simulink model "sim_all_2019b"  (R2019b)
settings: Solver=VariableStepAuto  StartTime=0.0  StopTime=2000  RelTol=1e-3
undefined symbols (not defined in the file or in its folder): a1, a2, alpha1, alpha2, cornerA, cornerB, cornerC, cornerD, ctrl_clockwise, ctrl_int_bound_or, ctrl_int_bound_pos, ctrl_k_or, ctrl_k_pos, ctrl_Ki_vel, ctrl_Kp_v_pos, ctrl_Kp_vel, ctrl_TAM, ctrl_Ts, ctrl_va_uncontrolled, ctrl_vel_uncontrolled, D, dead_zone_limit, depth, DiscIntNeverNeededParam, distanceFromWall, initInspectedSide, initPoint, mod_A, mod_Cd_F, mod_Cd_M, mod_eta_init, mod_g, mod_h0, mod_Ixx, mod_Iyy, mod_Izz, mod_Kp_dot, mod_lat0, mod_lon0, mod_m, mod_Mq_dot, mod_ni_init, mod_Nr_dot, mod_p1, mod_p2, mod_p3, mod_p4, mod_p5, mod_p6, mod_R, mod_Rm, mod_t1, mod_t2, mod_t3, mod_t4, mod_t5, mod_t6, mod_W, mod_Xu_dot, mod_Yv_dot ... (+53)
libraries: simulink x8, cstblocks x6, simulink_extras x1
(part 5 of 6)

== matlab function sim_all_2019b/Model/Vehicle Model/P3/Propeller3 ==
  data: n3 input; T3 output; V3 input; D parameter; omega parameter; a1 parameter; a2 parameter; alpha1 parameter; alpha2 parameter
function T3 = thrusterModel(n3, V3, D, omega, a1, a2, alpha1, alpha2)

Va3 = (1-omega) * V3;     % Advancement velocity at the propeller
J0 = Va3/(n3*D);          % Advancement Coefficient

if J0 > -alpha1/alpha2  % Out of linearity domain (right side)
    T3 = 0;              % A null generated thrust is assumed
    
elseif J0 < 0           % Out of linearity domain (left side)
    T3 = a1*abs(n3)*n3;    % Bollard thrust is assumed

else                    % Within the linearity domain
    T3 = a1*abs(n3)*n3 - a2*abs(n3)*V3;
end

== matlab function sim_all_2019b/Model/Vehicle Model/P4/Propeller4 ==
  data: n4 input; T4 output; V4 input; D parameter; omega parameter; a1 parameter; a2 parameter; alpha1 parameter; alpha2 parameter
function T4 = thrusterModel(n4, V4, D, omega, a1, a2, alpha1, alpha2)

Va4 = (1-omega) * V4;     % Advancement velocity at the propeller
J0 = Va4/(n4*D);          % Advancement Coefficient

if J0 > -alpha1/alpha2  % Out of linearity domain (right side)
    T4 = 0;              % A null generated thrust is assumed
    
elseif J0 < 0           % Out of linearity domain (left side)
    T4 = a1*abs(n4)*n4;    % Bollard thrust is assumed

else                    % Within the linearity domain
    T4 = a1*abs(n4)*n4 - a2*abs(n4)*V4;
end

== matlab function sim_all_2019b/Model/Vehicle Model/P5/Propeller5 ==
  data: n5 input; T5 output; V5 input; D parameter; omega parameter; a1 parameter; a2 parameter; alpha1 parameter; alpha2 parameter
function T5 = thrusterModel(n5, V5, D, omega, a1, a2, alpha1, alpha2)

Va5 = (1-omega) * V5;     % Advancement velocity at the propeller
J0 = Va5/(n5*D);          % Advancement Coefficient

if J0 > -alpha1/alpha2  % Out of linearity domain (right side)
    T5 = 0;              % A null generated thrust is assumed
    
elseif J0 < 0           % Out of linearity domain (left side)
    T5 = a1*abs(n5)*n5;    % Bollard thrust is assumed

else                    % Within the linearity domain
    T5 = a1*abs(n5)*n5 - a2*abs(n5)*V5;
end

== matlab function sim_all_2019b/Model/Vehicle Model/P6/Propeller6 ==
  data: n6 input; T6 output; V6 input; D parameter; omega parameter; a1 parameter; a2 parameter; alpha1 parameter; alpha2 parameter
function T6 = thrusterModel(n6, V6, D, omega, a1, a2, alpha1, alpha2)

Va6 = (1-omega) * V6;     % Advancement velocity at the propeller
J0 = Va6/(n6*D);          % Advancement Coefficient

if J0 > -alpha1/alpha2  % Out of linearity domain (right side)
    T6 = 0;              % A null generated thrust is assumed
    
elseif J0 < 0           % Out of linearity domain (left side)
    T6 = a1*abs(n6)*n6;    % Bollard thrust is assumed

else                    % Within the linearity domain
    T6 = a1*abs(n6)*n6 - a2*abs(n6)*V6;
end

== matlab function sim_all_2019b/Model/Vehicle Model/TAM ==
  data: T1 input; tau output; T2 input; T3 input; T4 input; T5 input; T6 input; eta input; mod_R parameter; mod_z_cm parameter
function tau = fcn (T1, T2, T3, T4, T5, T6, eta, mod_R, mod_z_cm)

% Si definisce il vettore delle forze e dei momenti applicati al veicolo al 
% variare dei propulsori immersi o emersi, si assume che i propulsori non 
% funzionino se utilizzati fuori dall'acqua. Si assume inoltre che il
% veicolo esca fuori dall'acqua orizzontalmente (con angoli di pitch e roll
% nulli).

z = eta(3);

% Veicolo completamente immerso, tutti i propulsori funzionano.
if (z >= (mod_R+mod_z_cm)) 
    tau1 = T1 + T2;
    tau2 = T3 + T4;
    tau3 = T5 + T6;
    tau4 = ((-(mod_R+mod_z_cm))*T3) + ((mod_R+mod_z_cm)*T4);
    tau5 = (-mod_R*T5) + (mod_R*T6);
    tau6 = (-mod_R*T1) + (mod_R*T2);
    
% Veicolo emerso in un range che va al dall'estremo superiore fino al 
% centro di massa (il centro di massa è ancora immerso), funzionano tutti i 
% propulsori tranne P4.
elseif (z >= 0 && z < (mod_R+mod_z_cm)) 
    tau1 = T1 + T2;
    tau2 = T3;
    tau3 = T5 + T6;
    tau4 = ((-(mod_R+mod_z_cm))*T3);
    tau5 = (-mod_R*T5) + (mod_R*T6);
    tau6 = (-mod_R*T1) + (mod_R*T2);

% Veicolo immerso in un range che va dall'estremo inferiore fino al centro 
% di massa (il centro di massa è emerso), funziona solo il propulsore P3.
elseif (z >= -(mod_R+mod_z_cm) && z < 0)
    tau1 = 0;
    tau2 = T3;
    tau3 = 0;
    tau4 = ((-(mod_R+mod_z_cm))*T3);
    tau5 = 0;
    tau6 = 0;

% Veicolo completamente emerso, nessun propulsore funziona.
else
    tau1 = 0;
    tau2 = 0;
    tau3 = 0;
    tau4 = 0;
    tau5 = 0;
    tau6 = 0;
end

tau = [tau1; tau2; tau3; tau4; tau5; tau6];

== matlab function sim_all_2019b/Model/Vehicle Model/Thruster Velocity Computation ==
  data: V1 output; V2 output; V3 output; V4 output; V5 output; V6 output; ni_rel input; mod_p1 parameter; mod_p2 parameter; mod_p3 parameter; mod_p4 parameter; mod_p5 parameter; mod_p6 parameter; mod_t1 parameter; mod_t2 parameter; mod_t3 parameter; mod_t4 parameter; mod_t5 parameter; mod_t6 parameter
function [V1, V2, V3, V4, V5, V6] = fcn(ni_rel, mod_p1, mod_p2, mod_p3, mod_p4, mod_p5, mod_p6, mod_t1, mod_t2, mod_t3, mod_t4, mod_t5, mod_t6)

% Si spezza il vettore velocità relativa nella componente lineare e angolare:
ni1_rel = [ni_rel(1); ni_rel(2); ni_rel(3)];
ni2_rel = [ni_rel(4); ni_rel(5); ni_rel(6)];

% Si definiscono i vettori velocità dei propulsori: 
Vp1 = ni1_rel + cross(ni2_rel, mod_p1);
Vp2 = ni1_rel + cross(ni2_rel, mod_p2);
Vp3 = ni1_rel + cross(ni2_rel, mod_p3);
Vp4 = ni1_rel + cross(ni2_rel, mod_p4);
Vp5 = ni1_rel + cross(ni2_rel, mod_p5);
Vp6 = ni1_rel + cross(ni2_rel, mod_p6);

% Si proiettano tali velocità lungo le direzioni date dai versori:
V1 = dot(Vp1, mod_t1); 
V2 = dot(Vp2, mod_t2);
V3 = dot(Vp3, mod_t3);
V4 = dot(Vp4, mod_t4);
V5 = dot(Vp5, mod_t5);
V6 = dot(Vp6, mod_t6);

== matlab function sim_all_2019b/Model/Vehicle Model/seaCurrent from NED to body ==
  data: seaCurrent_Velocity output; eta input; seaCurrent parameter
function seaCurrent_Velocity = fcn(eta, seaCurrent)

phi = eta(4);
theta = eta(5); 
psi = eta(6);

% Si definisce la matrice di rotazione J1 che mappa la velocità lineare 
% della corrente in terna body nella velocità lineare della corrente in 
% terna NED: 
J1 = [ cos(psi)*cos(theta)   -sin(psi)*cos(phi) + (cos(psi)*sin(theta)*sin(phi))   (sin(psi)*sin(phi)) + (cos(psi)*cos(phi)*sin(theta));
       sin(psi)*cos(theta)   (cos(psi)*cos(phi)) + (sin(psi)*sin(theta)*sin(phi))  (-cos(psi)*sin(phi)) + (sin(psi)*sin(theta)*cos(phi));
      -sin(theta)             cos(theta)*sin(phi)                                   cos(theta)*cos(phi)                                  ];

% Si definisce la matrice J1 inversa in maniera tale da mappare la velocità
% della corrente in terna NED nella velocità lineare della corrente in
% terna body (essendo J1 una matrice di rotazione l'inversa coincide con la
% trasposta):
J1_inv = J1';

%si definisce la velocità della corrente espressa in terna Body
seaCurrent_body = J1_inv*seaCurrent;
seaCurrent_Velocity = [seaCurrent_body; 0; 0; 0];

== matlab function sim_all_2019b/Model/from NED to ECEF ==
  data: eta1 input; eta1_ECEF output; mod_lat0 parameter; mod_lon0 parameter; mod_h0 parameter
function eta1_ECEF = fcn(eta1, mod_lat0, mod_lon0, mod_h0)

eta1_ECEF = [0; 0; 0];

eta1_North = eta1(1);
eta1_East = eta1(2);
eta1_Down = eta1(3);

coder.extrinsic('evalin','wgs84Ellipsoid','ned2geodetic')

[lat_ECEF, lon_ECEF, h_ECEF] = ned2geodetic(eta1_North, eta1_East, eta1_Down, mod_lat0, mod_lon0, mod_h0, wgs84Ellipsoid);

eta1_ECEF = [lat_ECEF; lon_ECEF; h_ECEF];

== matlab function sim_all_2019b/Sensors/BLOCCO GYRO1/Subsystem/GEOD to NED ==
  data: Bias_G output; t input
function Bias_G  = fcn(t)
ramp=t*(3.8785e-05);
Bias_G=ramp;

== matlab function sim_all_2019b/Controller_mk4_v3/C_pos/abs_integrator2/Body2Ned ==
  data: x_b input size=[3 1]; x_n output size=[3 1]; or input
%% Da BODY a NED per integrazione assoluta
function x_n = body2ned(x_b,or)
C=zeros(3,3);
C=Cx(or(1))'*Cy(or(2))'*Cz(or(3))';
x_n = C*x_b;
end

== matlab function sim_all_2019b/Controller_mk4_v3/C_pos/abs_integrator2/Ned2Body1 ==
  data: x_n input size=[3 1]; x_b output size=[3 1]; or input
%% Da NED a BODY
function x_b = ned2body(x_n,or)
C=zeros(3,3);
C=Cx(or(1))'*Cy(or(2))'*Cz(or(3))';
x_b = C'*x_n;
end

== matlab function sim_all_2019b/Controller_mk4_v3/C_pos/abs_integrator1/Body2Ned ==
  data: x_b input size=[3 1]; x_n output size=[3 1]; or input
%% Da BODY a NED
function x_n = body2ned(x_b,or)
C=zeros(3,3);
C=Cx(or(1))'*Cy(or(2))'*Cz(or(3))';
x_n = C*x_b;
end

== matlab function sim_all_2019b/Controller_mk4_v3/C_pos/abs_integrator1/Ned2Body1 ==
  data: x_n input size=[3 1]; x_b output size=[3 1]; or input
%% Da NED a BODY
function x_b = ned2body(x_n,or)
C=zeros(3,3);
C=Cx(or(1))'*Cy(or(2))'*Cz(or(3))';
x_b = C'*x_n;
end

== matlab function sim_all_2019b/Controller_mk4_v3/C_vel/abs_integrator/Body2Ned ==
  data: x_b input size=[3 1]; x_n output size=[3 1]; or input
%% Da BODY a NED
function x_n = body2ned(x_b,or)
C=zeros(3,3);
C=Cx(or(1))'*Cy(or(2))'*Cz(or(3))';
x_n = C*x_b;
end

== matlab function sim_all_2019b/Controller_mk4_v3/C_vel/abs_integrator/Ned2Body1 ==
  data: x_n input size=[3 1]; x_b output size=[3 1]; or input
%% Da NED a BODY
function x_b = ned2body(x_n,or)
C=zeros(3,3);
C=Cx(or(1))'*Cy(or(2))'*Cz(or(3))';
x_b = C'*x_n;
end

== matlab function sim_all_2019b/Mission_supervisor_v3/Mission_Supervisor/Risalita/MATLAB Function ==
  data: delta_SOS input; delta_current_ris output; delta_stato_ris output; Pos_d output size=3; Dpp_d output; Dps_d output; Pos_s input; Dpp_s input; Orp_s input; Dps_s input; distanceFromWall parameter; Orp_d output; relativeDirection parameter; soglia_pos parameter; SOS parameter; Dps_fin input; soglia_SOS_pos_ris parameter; soglia_SOS_orp parameter; error_flag input; SOS_205 input; initPoint parameter; soglia_SOS_collisione parameter
function [delta_current_ris, delta_stato_ris, Pos_d, Dpp_d, Dps_d, Orp_d ] = Risalita(delta_SOS, Pos_s, Dpp_s, Orp_s, Dps_s, distanceFromWall, relativeDirection, soglia_pos, SOS, Dps_fin, soglia_SOS_pos_ris, soglia_SOS_orp, error_flag, SOS_205, initPoint, soglia_SOS_collisione)

    disp("Risalita");
    
    %% Unità di misura 
    
    % Pos_d, Pos_s, soglia_pos, initPoint                                                                      [deg,deg,m]
    % Orp_d, Orp_s, soglia_SOS_orp                                                                             [rad]
    % relativeDirection                                                                                        [deg]
    % Dpp_d, Dps_d, Dpp_s, Dps_s, Dps_fin, distanceFromWall, soglia_SOS_collisione_s, soglia_SOS_collisione    [m]

    %% Inizializzazione variabili
    
    delta_stato_ris = 0;
    
    pronti = false; 
    
    %% Preparazione dei riferimenti da fornire ai blocchi successivi
    
    % Posizione da raggiungere
    Pos_d = [nan; nan; initPoint(3)];
    
    % Distanza da mantenere
    Dpp_d = distanceFromWall;
    Dps_d = Dps_fin;
    
    % Orientazione da mantenere
    Orp_d = deg2rad(relativeDirection);
    
    % Transizione di stato effettiva
    delta_current_ris = 301 - delta_SOS;  
    
    
    %% Verifica
    
    % Verifica sull'orientazione rispetto alla parete
    if (abs(Orp_s - Orp_d) > soglia_SOS_orp)
        
        SOS = 1;
        disp("EMERGENZA: Rilevato errore nell'orientazione relativa da parete");
        
    end
                                                                            %******TEST******
                                                                            %test = 30;
    % In base al meccanismo del "gestore dell'emergenza" si distinguono due casi: 
    % uno in cui lo stato di Risalita viene attivato al termine di un 
    % pattugliamento corretto (la codifica dello stato precedente è pari a 205) 
    % ed uno se la transizione in questo stato è dovuta all'aver
    % intrapreso una manovra di emergenza (lo stato precedente è
    % inferiore a 205).
    
    % Si proviene da un pattugliamento senza emergenza e si verifica di 
    % effettuare la risalita nella posizione giusta
    if (delta_SOS == 205 && SOS_205 == 0)
        if (abs(Dpp_s - Dpp_d) > soglia_SOS_pos_ris || ...                                          
            abs(Dps_s - Dps_fin) > soglia_SOS_pos_ris)
             
            SOS = 1;
            disp("EMERGENZA: Avvicinamento eccessivo alla parete");
            
        end
    
    % Si proviene da una situazione di emergenza oppure l'emergenza avviene in
    % "risalita". Verifica di effettuare la risalita senza collisione
    % con le pareti
    elseif (delta_SOS < 205 || SOS_205 == 1)
        
        if (abs(Dpp_s - Dpp_d) > soglia_SOS_collisione || ...
            abs(Dps_s) < soglia_SOS_collisione)
       
            SOS = 1;
            disp("EMERGENZA: Avvicinamento eccessivo alla parete");
            
        end
        
    end
    
    if error_flag == 1
        disp("EMERGENZA: Errore segnalato dagli altri sottosistemi");
        SOS = 1;
    end
    
                                                                            %*****TEST******% 
                                                                            %Dps_fin = 8;

    % Si verifica di aver raggiunto la superficie
    if (SOS == 0 && ... 
        abs(Pos_s(3) - Pos_d(3)) < soglia_pos(3)) 
    
          pronti = true;
        
    end
    
    
    %% Decisione dello stato successivo
    
    if ((pronti == true && (delta_SOS < 205 || SOS_205 == 1) || ...
        (SOS == 1)))
           
           delta_stato_ris = 304 - 301; % Transizione nello stato finale a causa di emergenza
    else
        if pronti == true
            
            delta_stato_ris = 302 - 301; % Transizione eseguita correttamente
        end
    end
    % Si rimane nello stato corrente
     
end

== matlab function sim_all_2019b/Controller_mk4_v3/lld2Ned1 ==
  data: x_ecef input size=[3 1]; x_n output; cornerC parameter
%% Da LLD (stima posizione assoluta) a NED
function x_n = ToNed_Pos(x_ecef,cornerC)
x_n=zeros(3,1);
coder.extrinsic('evalin', 'wgs84Ellipsoid', 'geodetic2ned');
[pNorth,pEast,pDown] = geodetic2ned(x_ecef(1),x_ecef(2),x_ecef(3),cornerC(1),cornerC(2),0,wgs84Ellipsoid);
x_n=[pNorth;pEast;x_ecef(3)];

end

== matlab function sim_all_2019b/Sensors/Environment and Sensors Model3/MATLAB Function1 ==
  data: pos input; plane_AB input; plane_BC input; plane_CD input; plane_DA input; plane_W input; dist output; Roll input; Pitch input; Yaw input
function dist = inter(pos,plane_AB,plane_BC,plane_CD,plane_DA,plane_W,Roll,Pitch, Yaw)
Nc=3; %numero di campioni per 'croce' di raggio del cono
WBr=deg2rad(5); % ampiezza semifascio del sonar (fascio considerato di 10°)
dist2=zeros(3,3);
R=linspace(Roll-WBr,Roll+WBr,Nc);
P=Pitch;
Y=linspace(Yaw-WBr, Yaw+WBr,Nc);
for j=1:Nc  %costruisco la croce (doppia)
for i=1:Nc
    
R_x = [1        0              0; %roll
      0 cos(R(i))  sin(R(i));
      0 -sin(R(i)) cos(R(i))];
  
R_y = [cos(P) 0 -sin(P); %pitch
          0           1         0;
       sin(P) 0 cos(P)];
   
R_z = [cos(Y(j)) sin(Y(j)) 0; %yaw
      -sin(Y(j)) cos(Y(j)) 0;
          0                 0        1];
      
jaco = (R_z'*R_y');
jacob = jaco*R_x';

    versore_son_body = [0 1 0]';
    versore_son_NED = jacob*versore_son_body;         %versore terna NED sonar prua

    %imposto il sistema per trovare l'intersezione tra la retta con direzione
    %nota e uno dei piani delle pareti del bacino

    t_AB = -(pos(1)+plane_AB(2)*pos(2)+plane_AB(4))/(plane_AB(2)*versore_son_NED(2)+versore_son_NED(1));
    t_BC = -(pos(1)+plane_BC(2)*pos(2)+plane_BC(4))/(plane_BC(2)*versore_son_NED(2)+versore_son_NED(1));
    t_CD = -(pos(1)+plane_CD(2)*pos(2)+plane_CD(4))/(plane_CD(2)*versore_son_NED(2)+versore_son_NED(1));
    t_DA = -(pos(1)+plane_DA(2)*pos(2)+plane_DA(4))/(plane_DA(2)*versore_son_NED(2)+versore_son_NED(1));
    t_W = -(plane_W(3)*pos(3)/(plane_W(3)*versore_son_NED(3)+versore_son_NED(3)));
    
    
    if t_AB < 0
        t_AB = inf;
    end
    if t_BC < 0
        t_BC = inf;
    end
    if t_CD < 0
        t_CD = inf;
    end
    if t_DA < 0
        t_DA = inf;
    end
    if t_W < 0
        t_W = inf;
    end
           dist1 = min([t_AB t_BC t_CD t_DA t_W]);
           
           if dist1==t_W %se incontro l'acqua metto NaN nella misura delle distanze
               dist2(i,j)=NaN;
           else
               dist2(i,j)=dist1;
           end
           
end
end
    contr=isnan(dist2); %controlla la presenza di NaN nel vettore di misure
    sum1=sum(sum(contr)); % conta il numero di NaN presenti
    
    if sum1>4 %incontro un numero di Nan superiore a 4
        dist=NaN;
    else
        dist=mean(nanmean(dist2));
    end
end

== matlab function sim_all_2019b/Sensors/Environment and Sensors Model4/MATLAB Function1 ==
  data: pos input size=[3]; plane_AB input; plane_BC input; plane_CD input; plane_DA input; plane_W input; dist output; Roll input; Pitch input; Yaw input
function dist = inter(pos,plane_AB,plane_BC,plane_CD,plane_DA,plane_W,Roll,Pitch, Yaw)
Nc=3; %numero di campioni per 'croce' di raggio del cono=1
WBr=deg2rad(5); % ampiezza semifascio del sonar (fascio considerato di 10°)
dist2=zeros(3,3);
R=linspace(Roll-WBr,Roll+WBr,Nc);
P=Pitch;
Y=linspace(Yaw-WBr, Yaw+WBr,Nc);
for j=1:Nc  %costruisco la croce (doppia)
for i=1:Nc
    
R_x = [1        0              0; %roll
      0 cos(R(i))  sin(R(i));
      0 -sin(R(i)) cos(R(i))];
  
R_y = [cos(P) 0 -sin(P); %pitch
          0           1         0;
       sin(P) 0 cos(P)];
   
R_z = [cos(Y(j)) sin(Y(j)) 0; %yaw
      -sin(Y(j)) cos(Y(j)) 0;
          0                 0        1];
      
jaco = (R_z'*R_y');
jacob = jaco*R_x';

    versore_son_body = [0 -1 0]';
    versore_son_NED = jacob*versore_son_body;         %versore terna NED sonar prua

    %imposto il sistema per trovare l'intersezione tra la retta con direzione
    %nota e uno dei piani delle pareti del bacino

    t_AB = -(pos(1)+plane_AB(2)*pos(2)+plane_AB(4))/(plane_AB(2)*versore_son_NED(2)+versore_son_NED(1));
    t_BC = -(pos(1)+plane_BC(2)*pos(2)+plane_BC(4))/(plane_BC(2)*versore_son_NED(2)+versore_son_NED(1));
    t_CD = -(pos(1)+plane_CD(2)*pos(2)+plane_CD(4))/(plane_CD(2)*versore_son_NED(2)+versore_son_NED(1));
    t_DA = -(pos(1)+plane_DA(2)*pos(2)+plane_DA(4))/(plane_DA(2)*versore_son_NED(2)+versore_son_NED(1));
    t_W = -(plane_W(3)*pos(3)/(plane_W(3)*versore_son_NED(3)+versore_son_NED(3)));
    
    
    if t_AB < 0
        t_AB = inf;
    end
    if t_BC < 0
        t_BC = inf;
    end
    if t_CD < 0
        t_CD = inf;
    end
    if t_DA < 0
        t_DA = inf;
    end
    if t_W < 0
        t_W = inf;
    end
           dist1 = min([t_AB t_BC t_CD t_DA t_W]);
           
           if dist1==t_W %se incontro l'acqua metto NaN nella misura delle distanze
               dist2(i,j)=NaN;
           else
               dist2(i,j)=dist1;
           end
           
end
end
    contr=isnan(dist2); %controlla la presenza di NaN nel vettore di misure
    sum1=sum(sum(contr)); % conta il numero di NaN presenti
    
    if sum1>4 %incontro un numero di Nan superiore a 4
        dist=NaN;
    else
        dist=mean(nanmean(dist2));
    end
end

== matlab function sim_all_2019b/Sensors/Environment and Sensors Model6/MATLAB Function1 ==
  data: pos input; plane_AB input; plane_BC input; plane_CD input; plane_DA input; plane_W input; dist output; Roll input; Pitch input; Yaw input
function dist = inter(pos,plane_AB,plane_BC,plane_CD,plane_DA,plane_W,Roll,Pitch, Yaw)
Nc=3; %numero di campioni per 'croce' di raggio del cono
WBr=deg2rad(5); % ampiezza semifascio del sonar (fascio considerato di 10°)
dist2=zeros(3,3);
R=Roll;
P=linspace(Pitch-WBr,Pitch+WBr,Nc);
Y=linspace(Yaw-WBr, Yaw+WBr,Nc);

for j=1:Nc  %costruisco la croce (doppia)
for i=1:Nc
    
R_x = [1        0              0; %roll
      0 cos(R)  sin(R);
      0 -sin(R) cos(R)];
  
R_y = [cos(P(i)) 0 -sin(P(i)); %pitch
          0           1         0;
       sin(P(i)) 0 cos(P(i))];
   
R_z = [cos(Y(j)) sin(Y(j)) 0; %yaw
      -sin(Y(j)) cos((j)) 0;
          0                 0        1];
      
jaco = (R_z'*R_y');
jacob = jaco*R_x';

    versore_son_body = [1 0 0]'; %prua
    versore_son_NED = jacob*versore_son_body;         %versore terna NED sonar prua

    %imposto il sistema per trovare l'intersezione tra la retta con direzione
    %nota e uno dei piani delle pareti del bacino

    t_AB = -(pos(1)+plane_AB(2)*pos(2)+plane_AB(4))/(plane_AB(2)*versore_son_NED(2)+versore_son_NED(1));
    t_BC = -(pos(1)+plane_BC(2)*pos(2)+plane_BC(4))/(plane_BC(2)*versore_son_NED(2)+versore_son_NED(1));
    t_CD = -(pos(1)+plane_CD(2)*pos(2)+plane_CD(4))/(plane_CD(2)*versore_son_NED(2)+versore_son_NED(1));
    t_DA = -(pos(1)+plane_DA(2)*pos(2)+plane_DA(4))/(plane_DA(2)*versore_son_NED(2)+versore_son_NED(1));
    t_W = -(plane_W(3)*pos(3)/(plane_W(3)*versore_son_NED(3)+versore_son_NED(3)));
    
    
    if t_AB < 0
        t_AB = inf;
    end
    if t_BC < 0
        t_BC = inf;
    end
    if t_CD < 0
        t_CD = inf;
    end
    if t_DA < 0
        t_DA = inf;
    end
    if t_W < 0
        t_W = inf;
    end
           dist1 = min([t_AB t_BC t_CD t_DA t_W]);
           
           if dist1==t_W %se incontro l'acqua metto NaN nella misura delle distanze
               dist2(i,j)=NaN;
           else
               dist2(i,j)=dist1;
           end
           
end
end
    contr=isnan(dist2); %controlla la presenza di NaN nel vettore di misure
    sum1=sum(sum(contr)); % conta il numero di NaN presenti
    
    if sum1>4 %incontro un numero di Nan superiore a 4
        dist=NaN;
    else
        dist=mean(nanmean(dist2));
    end
end

== matlab function sim_all_2019b/Sensors/Environment1 ==
  data: plane_AB output; plane_BC output; plane_CD output; plane_DA output; plane_W output
function [plane_AB,plane_BC,plane_CD,plane_DA,plane_W] = fcn()
%% Inizializzazione
% Coordinate degli spigoli del bacino in lat e long fornite dal file
% missionC.m
A= zeros(1,3);
B= zeros(1,3);
C= zeros(1,3);
D= zeros(1,3);
cornerA = [43.781381; 11.282793]; % Lat/Lon [decimal degrees]      
cornerB = [43.780975; 11.283505]; % Lat/Lon [decimal degrees]       
cornerC = [43.780189; 11.282698]; % Lat/Lon [decimal degrees]       
cornerD = [43.780602; 11.281956]; % Lat/Lon [decimal degrees]

% Definizione terna NED con origine (lat0,long0,h0) coincidente al 
% cornerD
coder.extrinsic('evalin', 'wgs84Ellipsoid', 'geodetic2ned');
lat0 = cornerC(1);
lon0 = cornerC(2);
h0 = 0;

%% Conversione ECEF to NED
[A(1),A(2),A(3)] = geodetic2ned(cornerA(1),cornerA(2),0,lat0,lon0,h0,wgs84Ellipsoid);
[B(1),B(2),B(3)] = geodetic2ned(cornerB(1),cornerB(2),0,lat0,lon0,h0,wgs84Ellipsoid);
[C(1),C(2),C(3)] = geodetic2ned(cornerC(1),cornerC(2),0,lat0,lon0,h0,wgs84Ellipsoid);
[D(1),D(2),D(3)] = geodetic2ned(cornerD(1),cornerD(2),0,lat0,lon0,h0,wgs84Ellipsoid);

%% Calcolo delle distanze dalle pareti
% L'equazione del piano corrisponde a quella della retta perché il piano
% delle pareti è verticale, per cui si risolve un sistema lineare:
% l'equazione del piano deve soddisfare il passaggio da due punti.
% Il parametro a è libero, lo poniamo a=1, il parametro c relativo all'asse
% z sarà sempre pari a zero.

% questo è il sistema da risolvere
b = - (B(1)- A(1)) /( B(2) - A(2) );   %AB
d = - A(1) - A(2)*b;

e = - (C(1)-B(1))/(C(2)-B(2));         %BC
f = - B(1) - B(2)*e;

g = - (D(1) - C(1)) / (D(2) - C(2));   %CD
h = - C(1) - C(2)*g;

i = - (A(1) - D(1))/(A(2) - D(2));     %DA
l = -D(1) - D(2)*i;

% syms b d;
% [b d] = solve(A(1)+b*A(2)+d,B(1)+b*B(2)+d,b,d);
a_AB = 1;
b_AB = double(b);
c_AB = 0;
d_AB = double(d);
% 
% syms b d ;
% [b d] = solve(B(1)+b*B(2)+d,C(1)+b*C(2)+d,b,d);
a_BC = 1;
b_BC = double(e);
c_BC = 0;
d_BC = double(f);

a_CD = 1;
b_CD = double(g);
c_CD = 0;
d_CD = double(h);

a_DA = 1;
b_DA = double(i);
c_DA = 0;
d_DA = double(l);


% calcolo dei coefficienti del piano direttamente con la formula esplicita
plane_AB = [a_AB b_AB c_AB d_AB];
plane_BC = [a_BC b_BC c_BC d_BC];
plane_CD = [a_CD b_CD c_CD d_CD];
plane_DA = [a_DA b_DA c_DA d_DA];
plane_W =[0 0 1 0];

== matlab function sim_all_2019b/Sensors/GEOD to NED1 ==
  data: z output; lat input; lon input; h input
function z  = fcn(lat,lon,h)
z=[0;0;0];
coder.extrinsic('evalin','wgs84Ellipsoid','geodetic2ned');
[N,E,D] = geodetic2ned(lat,lon,h,43.780189,11.282698,0,wgs84Ellipsoid);
z=[N;E;D];

== matlab function sim_all_2019b/Sensors/NED to GEOD1 ==
  data: z output; N input; E input
function z  = fcn(N,E)
z=zeros(2,1);
coder.extrinsic('evalin','wgs84Ellipsoid','ned2geodetic');
%profondità considerata come solo antenna GPS fuori dall'acqua
[LAT,LON,~]=ned2geodetic(N,E,-0.385,43.780189,11.282698,0,wgs84Ellipsoid);
z=[LAT;LON];

== matlab function sim_all_2019b/Model/from Rad to Deg ==
  data: eta2 input; eta2_deg output
function eta2_deg = fcn(eta2)

phi = eta2(1);
theta = eta2(2);
psi = eta2(3);

% Si effettua una conversione da radianti a gradi dell'angolo di roll:
k_phi = fix(phi/(2*pi));
orientation_phi = phi - (2*pi*k_phi);
phi_deg = (180*orientation_phi)/pi;

% Si effettua una conversione da radianti a gradi dell'angolo di pitch:
k_theta = fix(theta/(2*pi));
orientation_theta = theta - (2*pi*k_theta);
theta_deg = (180*orientation_theta)/pi;

% Si effettua una conversione da radianti a gradi dell'angolo di yaw:
k_psi = fix(psi/(2*pi));
orientation_psi = psi - (2*pi*k_psi);
psi_deg = (180*orientation_psi)/pi;

% Se si vuole mostrare anche il numero di rotazioni che compie il robot in
% roll, pitch o yaw mandare in uscita anche k_phi, k_theta e k_psi.

eta2_deg = [phi_deg; theta_deg; psi_deg];

== matlab function sim_all_2019b/Controller_mk4_v3/signal_to_NED/Signal_d->NED/ToNed ==
  data: vel input; ddp input; dps input; orp input; vel_n output size=[3 1]; wall_vect input; wall_vect2 input; state input; ctrl_clockwise parameter; ddp_n output size=[3 1]; dps_n output size=[3 1]; orp_n output size=[3 1]
%% A partire dai riferimenti scalari calcola i relativi vettori in terna NED
function [vel_n,ddp_n,dps_n,orp_n] = ToNed(vel, ddp, dps, orp, wall_vect, wall_vect2, state, ctrl_clockwise)
    w=wall_vect/norm(wall_vect);        % versore relativo alla pareta che stiamo pattugliando
    n = Cz(-pi/2)*wall_vect;            % vettore ortogonale entrante dalla parete in pattugliamento
    n=n/norm(n);                        % versore ortogonale alla parete in pattugliamento
    n2 = Cz(-pi/2)*wall_vect2;          % vettore ortogonale entrante dalla parete successiva
    n2=n2/norm(n2);                     % versore ortogonale alla parete successiva
    if ctrl_clockwise == true           % la velocità dipende dalla direzione di pattugliamento
        vel_n=w*vel;                    % stessa direzione della parete
    else
        vel_n=-w*vel;
    end
    ddp_n = n*ddp;                          % vettore distanza dalla parete in pattugliamento in ned
    dps_n = n2*dps;                         % vettore distanza dalla parete successiva in ned
    v_orp = -n;                             % deve essere uscente dal bacino
    v_orp = Cz(-orp)*v_orp;                 % ruoto dell' angolo di riferimento
    orp_n=[0;0;atan2(v_orp(2),v_orp(1))];   % angolo rispetto all'asse x della terna ned
    if(state == 203)                        % orp_n deve essere relativo alla parete successiva
        v_orp = -n2;
        v_orp = Cz(-orp)*v_orp;
        orp_n=[0;0;atan2(v_orp(2),v_orp(1))];
    end
end

== matlab function sim_all_2019b/Controller_mk4_v3/signal_to_NED/Signal_d->NED/wall_fcn ==
  data: wall_vect output; WALL input; cornerA parameter; cornerB parameter; cornerC parameter; cornerD parameter; wall_vect2 output; ctrl_clockwise parameter
%% Restituisce i vettori Parete in pattugliamento e Parete successiva
function [wall_vect, wall_vect2] = wall_fcn(WALL,cornerA, cornerB, cornerC, cornerD, ctrl_clockwise) %inspectionDirection
    AB = zeros(3,1);
    BC = zeros(3,1);
    CD = zeros(3,1);
    DA = zeros(3,1);
    a = zeros(3,1);
    b = zeros(3,1);
    c = zeros(3,1);
    d = zeros(3,1);
    coder.extrinsic('evalin', 'wgs84Ellipsoid', 'geodetic2ned');
    [aNorth,aEast,aDown] = geodetic2ned(cornerA(1),cornerA(2),0,cornerC(1),cornerC(2),0,wgs84Ellipsoid);
    [bNorth,bEast,bDown] = geodetic2ned(cornerB(1),cornerB(2),0,cornerC(1),cornerC(2),0,wgs84Ellipsoid);
    [cNorth,cEast,cDown] = geodetic2ned(cornerC(1),cornerC(2),0,cornerC(1),cornerC(2),0,wgs84Ellipsoid);
    [dNorth,dEast,dDown] = geodetic2ned(cornerD(1),cornerD(2),0,cornerC(1),cornerC(2),0,wgs84Ellipsoid);
    a=[aNorth;aEast;aDown];
    b=[bNorth;bEast;bDown];
    c=[cNorth;cEast;cDown];
    d=[dNorth;dEast;dDown];
    AB = b-a;
    BC = c-b;
    CD = d-c;
    DA = a-d;
    if WALL == 1
        wall_vect = AB;
        if ctrl_clockwise == true
            wall_vect2 = BC;
        else
            wall_vect2 = DA;
        end
    elseif WALL == 2
        wall_vect = BC;
        if ctrl_clockwise == true
            wall_vect2 = CD;
        else
            wall_vect2 = AB;
        end
    elseif  WALL == 3
        wall_vect = CD;
        if ctrl_clockwise == true
            wall_vect2 = DA;
        else
            wall_vect2 = BC;
        end
    else   
        wall_vect = DA;
        if ctrl_clockwise == true
            wall_vect2 = AB;
        else
            wall_vect2 = CD;
        end
    end
end

== matlab function sim_all_2019b/Controller_mk4_v3/C_or/eta_dot2ni ==
  data: eta_dot input; or input; va output
%% Da NED a BODY
function va = fcn(eta_dot, or)

phi= or(1);
theta= or(2); 
psi= or(3);

J2inv = [[1;0;0], Cx(phi)*[0;1;0], Cx(phi)*Cy(theta)*[0;0;1]];
va = J2inv * eta_dot;
end

== matlab function sim_all_2019b/Controller_mk4_v3/signal_to_NED/Signal_s->NED/ToNed ==
  data: ddp input; dps input; wall_vect input; ddp_n output size=[3 1]; dps_n output size=[3 1]; wall_vect2 input
%% A partire dalle stime scalari calcola i relativi vettori in terna NED
function [ddp_n,dps_n] = ToNed_s(ddp, dps,wall_vect, wall_vect2)
    n = Cz(-pi/2)*wall_vect;            % vettore ortogonale entrante dalla parete in pattugliamento
    n=n/norm(n);                        % versore ortogonale alla parete in pattugliamento
    n2 = Cz(-pi/2)*wall_vect2;          % vettore ortogonale entrante dalla parete successiva
    n2=n2/norm(n2);                     % versore ortogonale alla parete successiva
    ddp_n = n*ddp;                      % vettore distanza dalla parete in pattugliamento in ned
    dps_n = n2*dps;                     % vettore distanza dalla parete successiva in ned
end

== matlab function sim_all_2019b/Controller_mk4_v3/signal_to_NED/Signal_s->NED/wall_fcn1 ==
  data: wall_vect output; WALL input; cornerA parameter; cornerB parameter; cornerC parameter; cornerD parameter; wall_vect2 output; ctrl_clockwise parameter
%% Restituisce i vettori Parete in pattugliamento e Parete successiva
function [wall_vect, wall_vect2] = wall_fcn(WALL,cornerA, cornerB, cornerC, cornerD, ctrl_clockwise) %inspectionDirection
    AB = zeros(3,1);
    BC = zeros(3,1);
    CD = zeros(3,1);
    DA = zeros(3,1);
    a = zeros(3,1);
    b = zeros(3,1);
    c = zeros(3,1);
    d = zeros(3,1);
    coder.extrinsic('evalin', 'wgs84Ellipsoid', 'geodetic2ned');
    [aNorth,aEast,aDown] = geodetic2ned(cornerA(1),cornerA(2),0,cornerC(1),cornerC(2),0,wgs84Ellipsoid);
    [bNorth,bEast,bDown] = geodetic2ned(cornerB(1),cornerB(2),0,cornerC(1),cornerC(2),0,wgs84Ellipsoid);
    [cNorth,cEast,cDown] = geodetic2ned(cornerC(1),cornerC(2),0,cornerC(1),cornerC(2),0,wgs84Ellipsoid);
    [dNorth,dEast,dDown] = geodetic2ned(cornerD(1),cornerD(2),0,cornerC(1),cornerC(2),0,wgs84Ellipsoid);
    a=[aNorth;aEast;aDown];
    b=[bNorth;bEast;bDown];
    c=[cNorth;cEast;cDown];
    d=[dNorth;dEast;dDown];
    AB = b-a;
    BC = c-b;
    CD = d-c;
    DA = a-d;
    if WALL == 1
        wall_vect = AB;
        if ctrl_clockwise == true
            wall_vect2 = BC;
        else
            wall_vect2 = DA;
        end
    elseif WALL == 2
        wall_vect = BC;
        if ctrl_clockwise == true
            wall_vect2 = CD;
        else
            wall_vect2 = AB;
        end
    elseif  WALL == 3
        wall_vect = CD;
        if ctrl_clockwise == true
            wall_vect2 = DA;
        else
            wall_vect2 = BC;
        end
    else   
        wall_vect = DA;
        if ctrl_clockwise == true
            wall_vect2 = AB;
        else
            wall_vect2 = CD;
        end
    end
end

== matlab function sim_all_2019b/Controller_mk4_v3/signal_to_NED/prof_trigger ==
  settings: updateMethod=DISCRETE  sampleTime=ctrl_Ts
  data: state input; trigg_prof output
%% Trigger per la gestione dei segnali
% 1 se siamo in superficie
% 0 se siamo in profondità
function trigg_prof = fcn(state)
tmp = 0;
switch state
    case 100            % fermo in superficie
        tmp = 1;
    case 101            % orientazione verso parete di inizio in superficie
        tmp = 1;
    case 102            % posizionamento in superficie
        tmp = 1;   
    case 103            % immersione
        tmp = 1;
    case 104            % orientazione in profondità
        tmp = 0;
    case 201            % pattugliamento
        tmp = 0;
    case 202            % frenata
        tmp = 0;
    case 203            % manovra di cambio parete
        tmp = 0;
    case 204            % competamento del pattugliamento della parete iniziale
        tmp = 0;
    case 205            % frenata a metà parete
        tmp = 0;
    case 301            % risalita
        tmp = 0;
    case 302            % orientazione in superficie
        tmp = 1;
    case 303            % rientro, ritorno al punto iniziale in superficie
        tmp = 1;
    case 304            % fine missione, tutto spento
        tmp = 1;
end
trigg_prof = tmp;
end

== matlab function sim_all_2019b/Navigation/Calcolo distaza pareti/Calcolo distanza dalle pareti ==
  data: pos_es input; dpp output; dps output; parete_attuale input; nav_plane_AB parameter; nav_plane_BC parameter; nav_plane_CD parameter; nav_plane_DA parameter; nav_giro parameter
% Applicando la formula della distanza di un punto da un piano si ottiene la
% distanza della posizione dell'AUV dalla parete d'interesse. 

function [dpp,dps] = dpp_dps_calculator(pos_es, parete_attuale, nav_plane_AB, nav_plane_BC, nav_plane_CD, nav_plane_DA, nav_giro)
    
%selezione della parete di pattugliamento e successiva
    switch parete_attuale
        
        case 1
           coef = nav_plane_AB;            %parete attuale AB
           if nav_giro == 1
               coef_succ = nav_plane_BC;   %parete succ BC
           else
               coef_succ = nav_plane_DA;   %parete succ DA
           end
           
        case 2
           coef = nav_plane_BC;            %parete attuale BC
           if nav_giro == 1
               coef_succ = nav_plane_CD;   %parete succ CD
           else
               coef_succ = nav_plane_AB;   %parete succ AB
           end
           
        case 3
           coef = nav_plane_CD;            %parete attuale CD
           if nav_giro == 1
               coef_succ = nav_plane_DA;   %parete succ DA
           else
               coef_succ = nav_plane_BC;   %parete succ BC
           end
        case 4
           coef = nav_plane_DA;            %parete attuale DA
           if nav_giro == 1
               coef_succ = nav_plane_AB;   %parete succ AB
           else
               coef_succ = nav_plane_CD;   %parete succ CD
           end
        otherwise
            coef = [0 0 0 0];
            coef_succ = [0 0 0 0];
    end

    dpp = abs(coef(1)*pos_es(1)+coef(2)*pos_es(2)-coef(3)*pos_es(3)+coef(4))/norm([coef(1) coef(2) coef(3)]);
    dps = abs(coef_succ(1)*pos_es(1)+coef_succ(2)*pos_es(2)-coef_succ(3)*pos_es(3)+coef_succ(4))/norm([coef_succ(1) coef_succ(2) coef_succ(3)]);
   
end

== matlab function sim_all_2019b/Navigation/Calcolo distaza pareti/Calcolo orientazione dalla parete ==
  data: pos_es input; orient_parete output; parete_attuale input; orient input; nav_plane_AB parameter; nav_plane_BC parameter; nav_plane_CD parameter; nav_plane_DA parameter
function orient_parete  = orient_parete_calculator(pos_es, parete_attuale, orient, nav_plane_AB, nav_plane_BC, nav_plane_CD, nav_plane_DA)
    
    %consideriamo angoli di pitch e roll nulli, cioè si calcola
    %l'orientazione rispetto alla parete solo considerando rotazioni di yaw
    %(piano xy)

    Yaw   = orient(3);
    R_z = [cos(Yaw)     sin(Yaw)       0     ;
           -sin(Yaw)    cos(Yaw)       0     ;
              0            0           1    ];
    v_pos= R_z'*[1 0 0]';  %versore della retta lungo l'asse x (in body) in NED,
                       %cioè la direzione di riferimento di prua del veicolo     
    
    %selezione della parete di pattugliamento
switch parete_attuale                      
    case 1
        %% Piano di pattugliamento AB
        versore_plane_NED = [nav_plane_AB(1) nav_plane_AB(2) 0]';    %versore normale al piano
        versore_plane_NED = versore_plane_NED/norm(versore_plane_NED);

        %calcolo distanza e intersezione lungo la normale al piano
        t_ = -(pos_es(1)+nav_plane_AB(2)*pos_es(2)+nav_plane_AB(4))/(nav_plane_AB(2)*versore_plane_NED(2)+versore_plane_NED(1));
        inter_perp=zeros(3,1);
        inter_perp(1) = pos_es(1) + versore_plane_NED(1)*t_;
        inter_perp(2) = pos_es(2) + versore_plane_NED(2)*t_;
        inter_perp(3) = pos_es(3) + versore_plane_NED(3)*t_;
        
        %calcolo distanza e intersezione lungo la direzione di prua
        t_ = -(pos_es(1)+nav_plane_AB(2)*pos_es(2)+nav_plane_AB(4))/(nav_plane_AB(2)*v_pos(2)+v_pos(1));
        inter_prua=zeros(3,1);
        inter_prua(1) = pos_es(1) + v_pos(1)*t_;
        inter_prua(2) = pos_es(2) + v_pos(2)*t_;
        inter_prua(3) = pos_es(3) + v_pos(3)*t_;
        
        coef = nav_plane_AB;
        coef(4)=[];
        orient_parete = rad2deg(asin(abs(coef*v_pos)/(norm(coef)*norm(v_pos))));
        %se orient_parete è positiva, allora ci si trova tra - 90 e + 90 rispetto alla normale della parete 
        if t_ > 0              
            if inter_prua(1) > inter_perp(1) && inter_prua(2) < inter_perp(2)
                orient_parete = orient_parete - 90;
            else
                orient_parete = -(orient_parete - 90);
            end
        else
            if inter_prua(1) > inter_perp(1) && inter_prua(2) < inter_perp(2)
                orient_parete = (orient_parete + 90);
            else
                orient_parete = -(orient_parete + 90);
            end
        end    
    case 2
        %% Piano di pattugliamento BC
      	versore_plane_NED = [nav_plane_BC(1) nav_plane_BC(2) 0]';    %versore normale al piano
        versore_plane_NED = versore_plane_NED/norm(versore_plane_NED);

        %calcolo distanza e intersezione lungo la normale al piano
        t_ = -(pos_es(1)+nav_plane_BC(2)*pos_es(2)+nav_plane_BC(4))/(nav_plane_BC(2)*versore_plane_NED(2)+versore_plane_NED(1));
        inter_perp=zeros(3,1);
        inter_perp(1) = pos_es(1) + versore_plane_NED(1)*t_;
        inter_perp(2) = pos_es(2) + versore_plane_NED(2)*t_;
        inter_perp(3) = pos_es(3) + versore_plane_NED(3)*t_;

        %calcolo distanza e intersezione lungo la direzione di prua
        t_ = -(pos_es(1)+nav_plane_BC(2)*pos_es(2)+nav_plane_BC(4))/(nav_plane_BC(2)*v_pos(2)+v_pos(1));
        inter_prua=zeros(3,1);
        inter_prua(1) = pos_es(1) + v_pos(1)*t_;
        inter_prua(2) = pos_es(2) + v_pos(2)*t_;
        inter_prua(3) = pos_es(3) + v_pos(3)*t_;
        
        coef = nav_plane_BC;
        coef(4)=[];
        v_pos=-v_pos;
        orient_parete = rad2deg(asin(abs(coef*v_pos)/(norm(coef)*norm(v_pos))));
        %se orient_parete è positiva, allora ci si trova tra - 90 e + 90 rispetto alla normale della parete 
        if t_ > 0              
            if inter_prua(1) > inter_perp(1) && inter_prua(2) > inter_perp(2)
                orient_parete = orient_parete - 90;
            else
                orient_parete = -(orient_parete - 90);
            end
        else
            if inter_prua(1) > inter_perp(1) && inter_prua(2) > inter_perp(2)
                orient_parete = orient_parete + 90;
            else
                orient_parete = -(orient_parete + 90);
            end
        end
        
    case 3
        %% Piano di pattugliamento CD
      	versore_plane_NED = [nav_plane_CD(1) nav_plane_CD(2) 0]';    %versore normale al piano
        versore_plane_NED = versore_plane_NED/norm(versore_plane_NED);

        %calcolo distanza e intersezione lungo la normale al piano
        t_ = -(pos_es(1)+nav_plane_CD(2)*pos_es(2)+nav_plane_CD(4))/(nav_plane_CD(2)*versore_plane_NED(2)+versore_plane_NED(1));
        inter_perp=zeros(3,1);
        inter_perp(1) = pos_es(1) + versore_plane_NED(1)*t_;
        inter_perp(2) = pos_es(2) + versore_plane_NED(2)*t_;
        inter_perp(3) = pos_es(3) + versore_plane_NED(3)*t_;

        %calcolo distanza e intersezione lungo la direzione di prua
        t_ = -(pos_es(1)+nav_plane_CD(2)*pos_es(2)+nav_plane_CD(4))/(nav_plane_CD(2)*v_pos(2)+v_pos(1));
        inter_prua=zeros(3,1);
        inter_prua(1) = pos_es(1) + v_pos(1)*t_;
        inter_prua(2) = pos_es(2) + v_pos(2)*t_;
        inter_prua(3) = pos_es(3) + v_pos(3)*t_;
        
        coef = nav_plane_CD;
        coef(4)=[];
        v_pos=-v_pos;
        orient_parete = rad2deg(asin(abs(coef*v_pos)/(norm(coef)*norm(v_pos))));
        %se orient_parete è positiva, allora ci si trova tra - 90 e + 90 rispetto alla normale della parete 
        if t_ > 0              
            if inter_prua(1) > inter_perp(1) && inter_prua(2) < inter_perp(2)
                orient_parete = -orient_parete + 90;
            else
                orient_parete = orient_parete - 90;
            end
        else
             if inter_prua(1) > inter_perp(1) && inter_prua(2) < inter_perp(2)
                orient_parete = -orient_parete - 90;
            else
                orient_parete = orient_parete + 90;
            end
        end
        
    case 4
        %% Piano di pattugliamento DA
      	versore_plane_NED = [nav_plane_DA(1) nav_plane_DA(2) 0]';    %versore normale al piano
        versore_plane_NED = versore_plane_NED/norm(versore_plane_NED);

        %calcolo distanza e intersezione lungo la normale al piano
        t_ = -(pos_es(1)+nav_plane_DA(2)*pos_es(2)+nav_plane_DA(4))/(nav_plane_DA(2)*versore_plane_NED(2)+versore_plane_NED(1));
        inter_perp=zeros(3,1);
        inter_perp(1) = pos_es(1) + versore_plane_NED(1)*t_;
        inter_perp(2) = pos_es(2) + versore_plane_NED(2)*t_;
        inter_perp(3) = pos_es(3) + versore_plane_NED(3)*t_;

        %calcolo distanza e intersezione lungo la direzione di prua
        t_ = -(pos_es(1)+nav_plane_DA(2)*pos_es(2)+nav_plane_DA(4))/(nav_plane_DA(2)*v_pos(2)+v_pos(1));
        inter_prua=zeros(3,1);
        inter_prua(1) = pos_es(1) + v_pos(1)*t_;
        inter_prua(2) = pos_es(2) + v_pos(2)*t_;
        inter_prua(3) = pos_es(3) + v_pos(3)*t_;
        
        coef = nav_plane_DA;
        coef(4)=[];
        orient_parete = rad2deg(asin(abs(coef*v_pos)/(norm(coef)*norm(v_pos))));
        %se orient_parete è positiva, allora ci si trova tra - 90 e + 90 rispetto alla normale della parete 
        if t_ > 0              
            if inter_prua(1) < inter_perp(1) && inter_prua(2) < inter_perp(2)
                orient_parete = orient_parete - 90;
            else
                orient_parete = -orient_parete + 90;
            end
        else
            if inter_prua(1) < inter_perp(1) && inter_prua(2) < inter_perp(2)
                orient_parete = orient_parete + 90;
            else
                orient_parete = -orient_parete - 90;
            end
        end
        
    otherwise
        %%
       coef=[0 0 0 0];
       orient_parete = NaN;
end
    
    
end

== matlab function sim_all_2019b/Navigation/ECEF2NED ==
  data: GPS_ECEF input; GPS_NED output; nav_lat0 parameter; nav_lon0 parameter; nav_h0 parameter
%Componente di ingresso in terna ECEF
%Lat  [gradi]
%Long  [gradi]
%flag data_valid

function GPS_NED = GPS_conv_valid(GPS_ECEF, nav_lat0, nav_lon0, nav_h0)
    
    coder.extrinsic('evalin', 'wgs84Ellipsoid', 'geodetic2ned');

    if GPS_ECEF(3)==1
        GPS_NED = zeros(3,1);
        [GPS_NED(1),GPS_NED(2),GPS_NED(3)]= geodetic2ned(GPS_ECEF(1),GPS_ECEF(2),0,nav_lat0,nav_lon0,nav_h0,wgs84Ellipsoid);
        GPS_NED(3) = GPS_ECEF(3);
    else                            %qui non si effettua la conversione se il dato non è valido
        GPS_NED = GPS_ECEF; 
    end
end

== matlab function sim_all_2019b/Navigation/Extended Kalman Filter/AHRS__check/MATLAB Function4 ==
  data: flag_AHRS output; AHRS_new input; AHRS_now output; AHRS_old input
%gestione di misura errata di AHRS
function [flag_AHRS, AHRS_now] = fcn(AHRS_new, AHRS_old)

    if isnan(AHRS_new(1,1)) || isnan(AHRS_new(2,1)) || isnan(AHRS_new(3,1))
        AHRS_now = AHRS_old;
        flag_AHRS = 1;
        disp('Misura AHRS non valida')
    else
        AHRS_now = AHRS_new;
        flag_AHRS = 0;
    end  
end

== matlab function sim_all_2019b/Navigation/Extended Kalman Filter/CORREZIONE/MATLAB Function ==
  data: x_k_k_1 input; x_k output; P_k_k_1 input; e input size=6 1; H input size=6 3; R_k input size=6 6; P_k output; nav_flag_init input
%%Passo di Correzione

function [x_k, P_k] = correction(x_k_k_1,P_k_k_1, e, H, R_k,nav_flag_init)
    
     x_k = zeros(3,1);
     P_k = zeros(3,3);
     
     
    if nav_flag_init ~= 0
        %matrice ottenuta da derivata di funzione h (6x1) per i rumori sei vari
        %sensori, che sono 6. (ha dimensione 6x6)
        %andrebbero anche considerati i rumori legati all'AHRS che al momento
        %sono trascurati
        %M = eye(6,6);              %M è l'dientità
        S_k = H*P_k_k_1*H'+ R_k;
        K_k = P_k_k_1*H'*(inv(S_k));

        P_k = (eye(3)-(K_k*H))*P_k_k_1;
        x_k = x_k_k_1 + K_k * e;
    end

end
